simulink model "DT_DSM_THIRD_ORDER_OSR_2048"  (R2025b)
settings: Solver=VariableStepAuto  StartTime=0.0  StopTime=5  RelTol=1e-3
undefined symbols (not defined in the file): dspblkCoreblockFVToolHelper, gcbh
libraries: simulink_extras x1
settings Model: Creator=Team_33  LastModifiedBy=k2vas

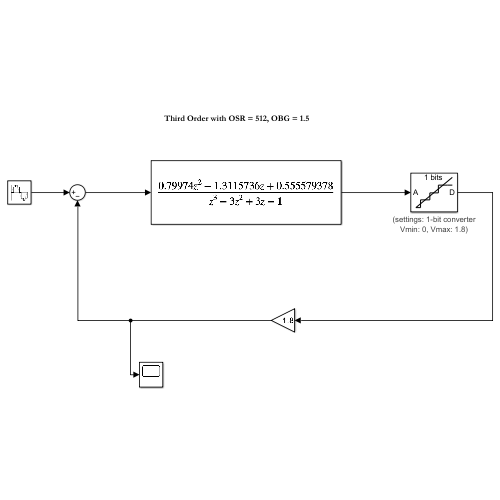
[thumbnail: Simulink's stored preview of the top-level diagram]
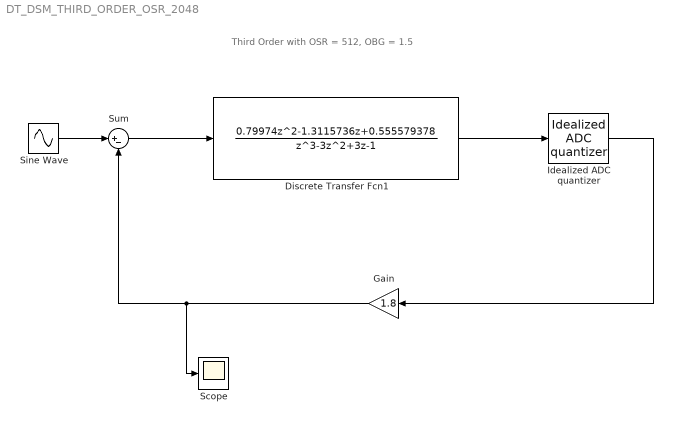
== system DT_DSM_THIRD_ORDER_OSR_2048 ==
  note: Third Order with OSR = 512, OBG = 1.5
  Discrete Transfer Fcn1 : DiscreteTransferFcn  LoadFcn=dspblkCoreblockFVToolHelper(gcbh,'load');  Numerator=[0.79974 -1.3115736 0.555579378]  Denominator=[1 -3 3 -1]
      settings: CopyFcn=dspblkCoreblockFVToolHelper(gcbh,'copy');  DeleteFcn=dspblkCoreblockFVToolHelper(gcbh,'close');  ModelCloseFcn=dspblkCoreblockFVToolHelper(gcbh,'close');  PreSaveFcn=dspblkCoreblockFVToolHelper(gcbh,'presave');  PostSaveFcn=dspblkCoreblockFVToolHelper(gcbh,'postsave');  CloseFcn=dspblkCoreblockFVToolHelper(gcbh,'close');
  Gain : Gain  Gain=1.8
  Idealized ADC quantizer : simulink_extras/Additional Discrete/Idealized ADC quantizer  NumberOfConverterBits=1  Vmin=0  Vmax=1.8  OutputDataType=int32  OutputNegativeValues=off
  Scope : Scope
      settings: ActiveDisplayYMinimum=0.17302  ActiveDisplayYMaximum=0.7879  DataLoggingVariableName=output_data  DataLoggingSaveFormat=Array
  Sine Wave : Sin  Amplitude=0.6  Bias=0.9  Frequency=((2000*512)*127*4*2*pi)/(32768*32)  SampleTime=1/(2000*512)
  Sum : Sum  Inputs=|+-
  wires:
  Idealized ADC quantizer/1 -> Gain/1
  Discrete Transfer Fcn1/1 -> Idealized ADC quantizer/1
  Sum/1 -> Discrete Transfer Fcn1/1
  Sine Wave/1 -> Sum/1
  Gain/1 -> Scope/1, Sum/2
